simulink model "d5_b_1_model"  (R2025a)
settings: Solver=VariableStepAuto  StartTime=0.0  StopTime=10.0  RelTol=1e-3
values from neighbouring files (symbols this model uses):
  A = Gp.Denominator{1,1}    [d5_RST.m]    (also in d5_a_1.m = Gpk.Denominator{1,1}; d5_a_2.m = Gpk.Denominator{1,1}; d5_b_1.m = Gpd.Denominator{1,1})
  B = Gp.Numerator{1,1}    [d5_RST.m]    (also in d5_a_1.m = Gpk.Numerator{1,1}; d5_a_2.m = Gpk.Numerator{1,1}; d5_b_1.m = Gpd.Numerator{1,1})
  Rd = [1, RS(1) - 1, -RS(1)]    [d5_b_1.m]
  Sd = RS(2:end)'    [d5_b_1.m]
  Ts = 0.001    [d5_b_1.m]    (also in d5_b_2.m)
  Tsd = 1 / dcgain(minreal(1/Rsd * feedback(Gpd, Ssd/Rsd)))    [d5_b_1.m]
settings Model: Creator=Korisnik  LastModifiedBy=Korisnik

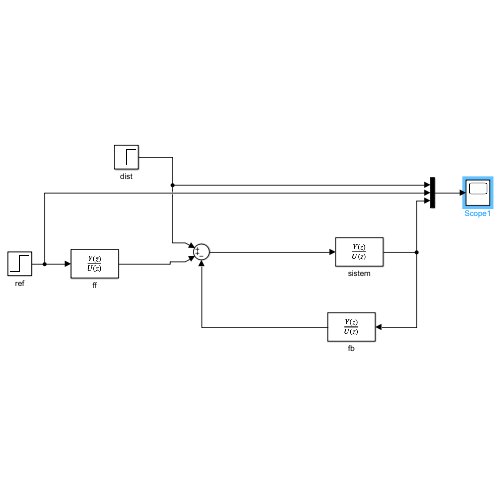
[thumbnail: Simulink's stored preview of the top-level diagram]
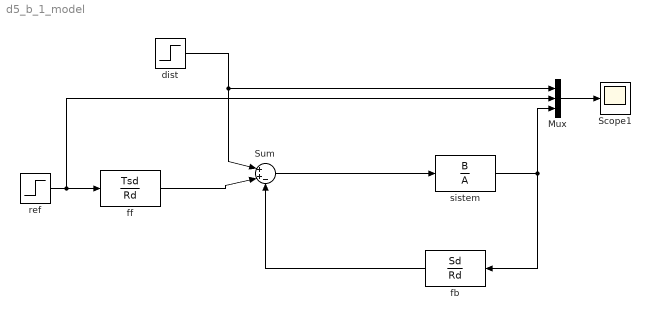
== system d5_b_1_model ==
  Mux : Mux  Inputs=3
  Scope1 : Scope
      settings: ActiveDisplayYMinimum=0.26691094826257533  ActiveDisplayYMaximum=11.698531433899923
  Sum : Sum  Inputs=|++-
  dist : Step  Time=3  After=4  SampleTime=0
  fb : DiscreteTransferFcn  Numerator=Sd  Denominator=Rd
  ff : DiscreteTransferFcn  Numerator=Tsd  Denominator=Rd
  ref : Step  Time=0  After=8  SampleTime=Ts
  sistem : DiscreteTransferFcn  Numerator=B  Denominator=A
  wires:
  ref/1 -> Mux/2, ff/1
  sistem/1 -> Mux/3, fb/1
  ff/1 -> Sum/2
  dist/1 -> Sum/1, Mux/1
  fb/1 -> Sum/3
  Sum/1 -> sistem/1
  Mux/1 -> Scope1/1
